simulink model "simulation_ex10"  (R2023a)
settings: Solver=VariableStepAuto  StartTime=0.0  StopTime=20  RelTol=1e-3
values from neighbouring files (symbols this model uses):
  D = sqrt(D)    [ex03.m]    (also in ex05.m = [0; 0]; ex10.m = 0.1; ex11.m = 0; ex11_2.m = [0 0; 0 1])
  M = 1    [ex10.m]
settings Model: Creator=vigro  LastModifiedBy=vigro

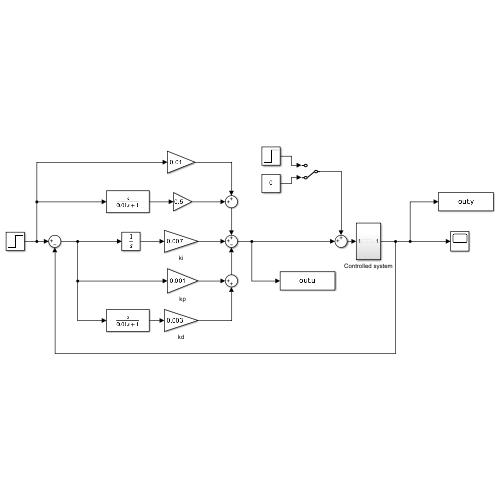
[thumbnail: Simulink's stored preview of the top-level diagram]
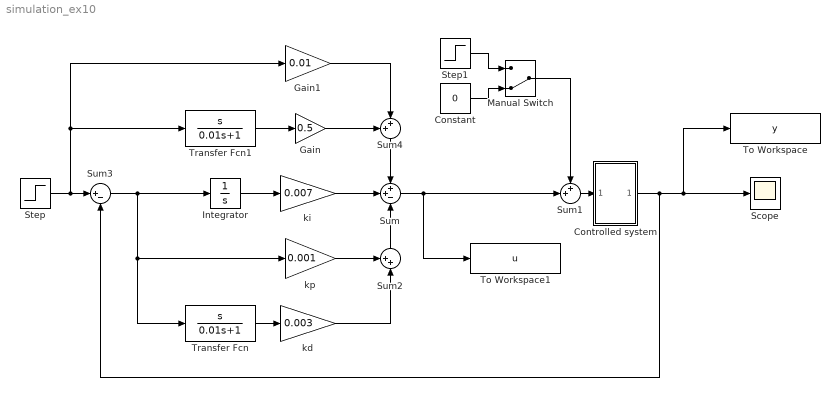
== system simulation_ex10 ==
  Constant : Constant  Value=0
  Controlled system : Subsystem
  Gain : Gain  Gain=0.5
  Gain1 : Gain  Gain=0.01
  Integrator : Integrator
  Manual Switch : ManualSwitch  CurrentSetting=0
  Scope : Scope
  Step : Step  Time=0  SampleTime=0
  Step1 : Step  SampleTime=0
  Sum : Sum  Inputs=++-
  Sum1 : Sum  Inputs=++|
  Sum2 : Sum  Inputs=++|
  Sum3 : Sum  Inputs=|+-
  Sum4 : Sum  Inputs=++|
  To Workspace : ToWorkspace  VariableName=y  SaveFormat=Timeseries  SampleTime=-1
  To Workspace1 : ToWorkspace  VariableName=u  SaveFormat=Timeseries  SampleTime=-1
  Transfer Fcn : TransferFcn  Numerator=[1 0]  Denominator=[0.01 1]
  Transfer Fcn1 : TransferFcn  Numerator=[1 0]  Denominator=[0.01 1]
  kd : Gain  Gain=0.003
  ki : Gain  Gain=0.007
  kp : Gain  Gain=0.001
  wires:
  Sum1/1 -> Controlled system/1(In1)
  Sum/1 -> To Workspace1/1, Sum1/2
  kp/1 -> Sum2/1
  kd/1 -> Sum2/2
  Integrator/1 -> ki/1
  Transfer Fcn/1 -> kd/1
  Step/1 -> Gain1/1, Transfer Fcn1/1, Sum3/1
  Sum3/1 -> Transfer Fcn/1, kp/1, Integrator/1
  Controlled system/1(Out1) -> Scope/1, To Workspace/1, Sum3/2
  Step1/1 -> Manual Switch/1
  Constant/1 -> Manual Switch/2
  Manual Switch/1 -> Sum1/1
  ki/1 -> Sum/2
  Sum2/1 -> Sum/3
  Gain/1 -> Sum4/1
  Gain1/1 -> Sum4/2
  Sum4/1 -> Sum/1
  Transfer Fcn1/1 -> Gain/1

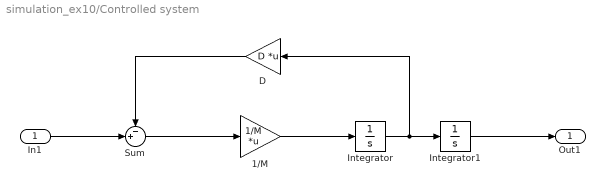
== system simulation_ex10/Controlled system ==
  In1 : Inport
  1/M : Gain  Gain=1/M  Multiplication=Matrix(K*u) (u vector)
  D : Gain  Gain=D  Multiplication=Matrix(K*u) (u vector)
  Integrator : Integrator
  Integrator1 : Integrator
  Sum : Sum  Inputs=-+|
  Out1 : Outport
  wires:
  D/1 -> Sum/1
  Integrator/1 -> D/1, Integrator1/1
  1/M/1 -> Integrator/1
  Sum/1 -> 1/M/1
  In1/1 -> Sum/2
  Integrator1/1 -> Out1/1
